simulink model "SHM_900HZ_TG190428test"  (Simulink 7.7)
settings: Solver=ode113  SolverMode=SingleTasking  StartTime=0.0  StopTime=3  RelTol=0.5e-4
undefined symbols (not defined in the file): D11, Delta, SHM900
libraries: powerlib x37, powerlib_extras x22, simulink x6, simulink_extras x1
(part 1 of 2)
settings Model: Creator=wufenglin  LastModifiedBy=jinxuefeng  SimulationMode=accelerator
settings SolverCC: AutoInsertRateTranBlk=on
settings OptimizationCC: InitFltsAndDblsToZero=on  EfficientMapNaN2IntZero=off
settings DebuggingCC: SaveWithParameterizedLinksMsg=none  SignalResolutionControl=TryResolveAllWithWarning  UnconnectedInputMsg=none  UnconnectedOutputMsg=none  UnconnectedLineMsg=none  StrictBusMsg=Warning
settings HardwareCC: TargetIntDivRoundTo=Zero  TargetEndianess=LittleEndian  TargetHWDeviceType=MATLAB Host  ProdEqTarget=off
settings CodeAppCC: MaxIdLength=128

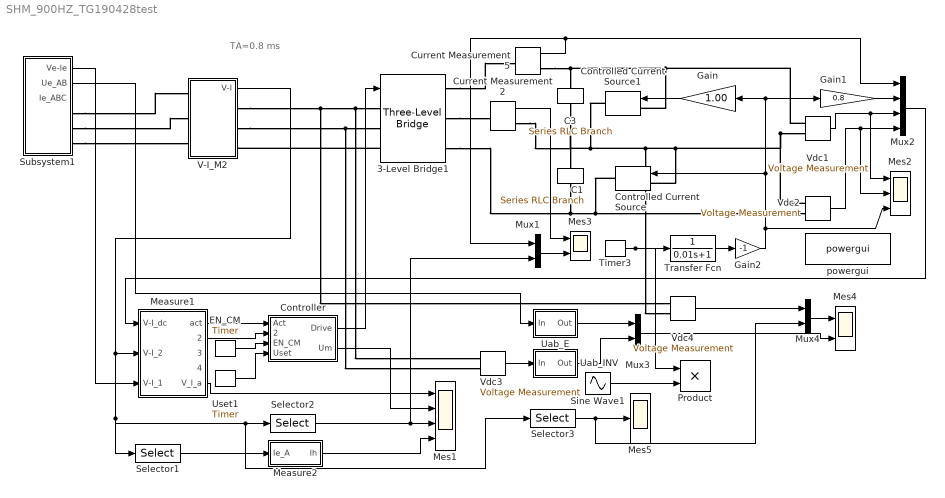
== system SHM_900HZ_TG190428test ==
  note: TA=0.8 ms
  3-Level Bridge1 : powerlib/Power Electronics/Three-Level Bridge  SystemSampleTime=-1  Arms=3  SnubberResistance=10000  SbubberCapacitance=1e-6  Device=MOSFET / Diodes  Ron=0.2e-3  ForwardVoltages="[  2 1 ]"  Measurements=None
  C1 : powerlib/Elements/Series RLC Branch  PhysicalDomain=powersysdomain  SubClassName=unknown  LeftPortType=p1  RightPortType=p1  LConnTagsString=__new0  RConnTagsString=__new0  BranchType=C  Resistance=1.0  Inductance=1.0  SetiL0=off  InitialCurrent=0  Capacitance=14e-3  Setx0=on  InitialVoltage=2600  Measurements=None
  C3 : powerlib/Elements/Series RLC Branch  PhysicalDomain=powersysdomain  SubClassName=unknown  LeftPortType=p1  RightPortType=p1  LConnTagsString=__new0  RConnTagsString=__new0  BranchType=C  Resistance=1.0  Inductance=1.0  SetiL0=off  InitialCurrent=0  Capacitance=14e-3  Setx0=on  InitialVoltage=2600  Measurements=None
  Controlled Current Source : powerlib/Electrical Sources/Controlled Current Source  SystemSampleTime=-1  Initialize=on  Source_Type=AC  Amplitude=0  Phase=0  Frequency=0  Measurements=None
  Controlled Current Source1 : powerlib/Electrical Sources/Controlled Current Source  SystemSampleTime=-1  Initialize=on  Source_Type=AC  Amplitude=0  Phase=0  Frequency=0  Measurements=None
  Controller : Subsystem  mask{Ts=1e-6, TA=1/1800, fn=50, Kp_v=3, Tn_v=0.2, Kp_I=0.1, Tn_I=0.05, K1=1.011, T1=0.005, Iq0=-0.278*0, La=0.23, Td=2.5e-5, U2=3.3, Kpre=5, Kp_v_scal=2}
      mask prompts: Ts "Ts [s]"; TA "TA [s]"; fn "fn [Hz]"; T1 "T1 [s]"
  Current Measurement2 : powerlib/Measurements/Current Measurement  SystemSampleTime=-1  PhasorSimulation=off  OutputType=Complex  PSBequivalent=0
  Current Measurement5 : powerlib/Measurements/Current Measurement  SystemSampleTime=-1  PhasorSimulation=off  OutputType=Complex  PSBequivalent=0
  EN_CM : powerlib_extras/Control  Blocks/Timer  SystemSampleTime=-1  t="[ 0  10]"  e="[1  1]"
  Gain : Gain  Gain=1.00
  Gain1 : Gain  Gain=0.8
  Gain2 : Gain  Gain=-1
  Measure1 : Subsystem  mask{Ts=1e-6, TA=1/1800, Sn=8, U1=10, U2=3.3, Udc=2.4}
      mask prompts: Ts "Ts [s}"; TA "TA [s]"; Sn "Sn [MVA]"; U1 "U1 [kV]"; U2 "U2 [kV]"; Udc "Udc [kV]"
  Measure2 : Subsystem
  Mes1 : Scope  NumInputPorts=4
      settings: YMin=-1.1~-5~-5~-5  YMax=1.1~5~5~5  SaveName=Vdc2  SampleInput=on  SampleTime=1e-5
  Mes2 : Scope  NumInputPorts=3
      settings: YMin=2399.85~2399.84~-5  YMax=2399.89~2399.89~5  SaveName=Vdc  DataFormat=Array  SampleInput=on  SampleTime=1e-5
  Mes3 : Scope  NumInputPorts=2
      settings: YMin=-1.1~-5  YMax=1.1~5  SaveName=Vdc1  DataFormat=Array  SampleInput=on  SampleTime=1e-5
  Mes4 : Scope  NumInputPorts=2
      settings: YMin=-1000~-5  YMax=4750~5  SaveName=Vdc4  DataFormat=Array  SampleInput=on  SampleTime=1e-5
  Mes5 : Scope
      settings: YMin=-1.1  YMax=1.1  SaveName=IA_SHM900  SampleInput=on  SampleTime=1e-5
  Mux1 : Mux  Inputs=2
  Mux2 : Mux
  Mux3 : Mux  Inputs=2
  Mux4 : Mux  Inputs=2
  Product : Product  RndMeth=Zero
  Selector1 : Selector  InputPortWidth=5  IndexOptions=Index vector (dialog)  Indices=3  OutputSizes=1
  Selector2 : Selector  InputPortWidth=5  IndexOptions=Index vector (dialog)  Indices=[3 4 5]  OutputSizes=1
  Selector3 : Selector  InputPortWidth=5  IndexOptions=Index vector (dialog)  Indices=3  OutputSizes=1
  Sine Wave1 : Sin  Amplitude=0.8  Frequency=4*pi  SampleTime=0
  Subsystem1 : Subsystem
  Timer3 : powerlib_extras/Control  Blocks/Timer  SystemSampleTime=-1  t="[ 0  0.6 1.1 1.3]"  e="[0  1200  1200 1200]"
  Transfer Fcn : TransferFcn  Denominator=[0.01 1]
  Uab_E : Subsystem  mask{Period=0.667e-3, buf=2048}
      mask prompts: Period "average period"; buf "buffer size"
  Uab_INV : Subsystem  mask{Period=0.667e-3, buf=2048}
      mask prompts: Period "average period"; buf "buffer size"
  Uset1 : powerlib_extras/Control  Blocks/Timer  SystemSampleTime=-1  t="[ 0  10]"  e="[1.08  1]"
  V-I_M2 : Subsystem
  Vdc{1..4} (4 alike) : powerlib/Measurements/Voltage Measurement  Tag=PoWeRsYsTeMmEaSuReMeNt  SystemSampleTime=-1  PhasorSimulation=off  OutputType=Magnitude  PSBequivalent=0
  powergui : powerlib/powergui  SystemSampleTime=-1  SimulationMode=Discrete  SampleTime=1e-6  frequency=60  SPID=off  DisableSnubberDevices=off  DisableRonSwitches=off  DisableVfSwitches=off  SwTol=0  Interpol=off  DisplayEquations=off  FunctionMessages=off  frequencyindice=0  Pbase=100e6  ErrMax=1e-4  Iterations=50  UnitsV=kV  UnitsW=MW  echomessages=off  HookPort=off  EnableUseOfTLC=off  x0status=blocks  RestoreLinks=warning  ResistiveCurrentMeasurement=off  Frange=[0:2:500]  Ylog=off  Xlog=on  ShowGrid=off  save=off  variable=ZData  structure=IA_SHM900  ZoomFFT=off  StartTime=0.6  cycles=20  DisplayStyle=1  fundamental=50  FreqAxis=on  MaxFrequency=2000  frequencyindicesteady=1  RmsSteady=1  display=off  Ts=0  methode=off
  wires:
  Vdc2/1 -> Mux2/4, Mes2/2
  Mux2/1 -> Measure1/1(V-I_dc)
  Vdc1/1 -> Mux2/3, Mes2/1
  Current Measurement5/1 -> Mux2/1, Mux1/1
  Measure1/1(act) -> Controller/1(Act)
  Transfer Fcn/1 -> Gain2/1
  Controller/1(Drive) -> 3-Level Bridge1/1
  Mux1/1 -> Mes3/2
  Current Measurement2/1 -> Mes3/1
  V-I_M2/1(V-I) -> Measure1/2(V-I_2), Selector1/1, Selector2/1, Selector3/1
  Measure1/5(V_I_a) -> Mes1/1
  Uab_E/1(Out) -> Mux3/1
  Uab_INV/1(Out) -> Mux3/2
  Vdc3/1 -> Uab_INV/1(In)
  Measure1/2(Vdc_sub) -> Controller/2(Udc_sub)
  Gain/1 -> Controlled Current Source1/1
  EN_CM/1 -> Controller/3(EN_CM)
  Selector2/1 -> Mes1/3, Mux1/2
  Subsystem1/1(Ve-Ie) -> Measure1/3(V-I_1)
  Subsystem1/2(Ue_AB) -> Uab_E/1(In)
  Measure2/1(Ih) -> Mes1/4
  Selector1/1 -> Measure2/1(Ie_A)
  Selector3/1 -> Mes5/1, Mux4/2
  Controller/2(Um) -> Mes1/2
  Mux3/1 -> Mes4/2
  Uset1/1 -> Controller/4(Uset)
  Timer3/1 -> Product/1, Transfer Fcn/1
  Vdc4/1 -> Mux4/1
  Mux4/1 -> Mes4/1
  Gain1/1 -> Mux2/2
  Sine Wave1/1 -> Product/2
  Gain2/1 -> Controlled Current Source/1, Gain/1, Gain1/1, Mes2/3
  connections:
  Vdc1/LConn1 -- Current Measurement5/RConn1 -- C3/LConn1 -- Controlled Current Source1/LConn1
  3-Level Bridge1/RConn1 -- Current Measurement5/LConn1
  V-I_M2/RConn1 -- 3-Level Bridge1/LConn1 -- Vdc3/LConn1 -- Vdc4/LConn1
  V-I_M2/RConn2 -- 3-Level Bridge1/LConn2 -- Vdc3/LConn2
  3-Level Bridge1/LConn3 -- V-I_M2/RConn3
  3-Level Bridge1/RConn2 -- Current Measurement2/LConn1
  Vdc2/LConn1 -- Vdc1/LConn2 -- Controlled Current Source/LConn1 -- Current Measurement2/RConn1 -- C1/LConn1 -- C3/RConn1 -- Controlled Current Source1/RConn1 -- Vdc4/LConn2
  3-Level Bridge1/RConn3 -- C1/RConn1 -- Vdc2/LConn2 -- Controlled Current Source/RConn1
  Subsystem1/RConn3 -- V-I_M2/LConn3
  Subsystem1/RConn2 -- V-I_M2/LConn2
  Subsystem1/RConn1 -- V-I_M2/LConn1

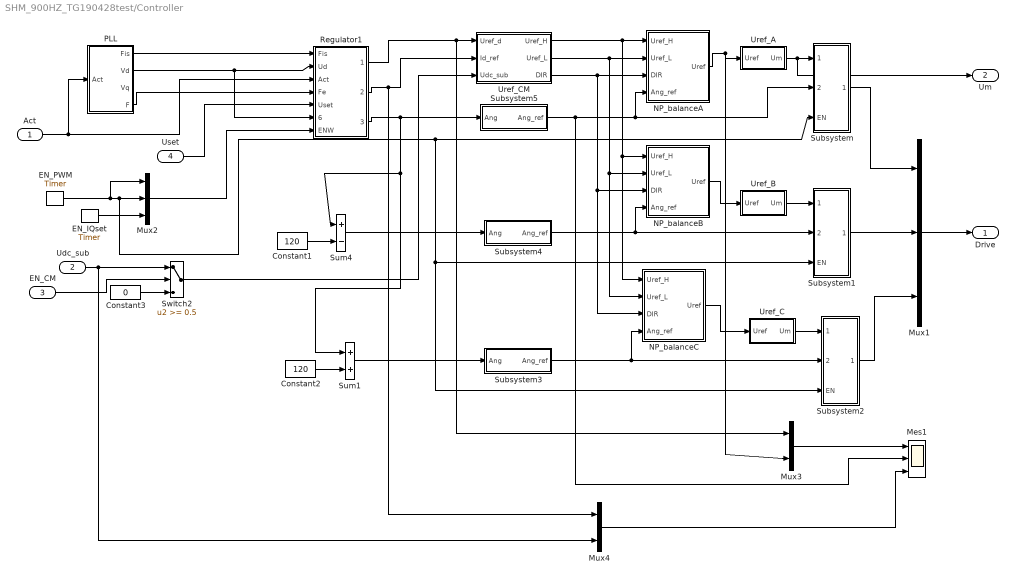
== system SHM_900HZ_TG190428test/Controller ==
  Act : Inport
  Udc_sub : Inport  Port=2
  EN_CM : Inport  Port=3
  Uset : Inport  Port=4
  Constant1 : Constant  Value=120
  Constant2 : Constant  Value=120
  Constant3 : Constant  Value=0
  EN_IQset : powerlib_extras/Control  Blocks/Timer  SystemSampleTime=-1  t="[ 0    0.16  0.22 ]"  e="[  0  1  1]"
  EN_PWM : powerlib_extras/Control  Blocks/Timer  SystemSampleTime=-1  t="[ 0    0.1 ]"  e="[  0  1 ]"
  Mes1 : Scope  NumInputPorts=3
      settings: YMin=-1.1~-5~-5  YMax=1.1~5~5  SaveName=Vdc6  SampleInput=on  SampleTime=1e-5
  Mux1 : Mux  Inputs=3
  Mux2 : Mux  Inputs=3
  Mux3 : Mux  Inputs=2
  Mux4 : Mux  Inputs=2
  NP_balanceA : Subsystem
  NP_balanceB : Subsystem
  NP_balanceC : Subsystem
  PLL : Subsystem
  Regulator1 : Subsystem
  Subsystem : Subsystem
  Subsystem1 : Subsystem
  Subsystem2 : Subsystem
  Subsystem3 : Subsystem
  Subsystem4 : Subsystem
  Subsystem5 : Subsystem
  Sum1 : Sum  SampleTime=Ts
  Sum4 : Sum  Inputs=+-  SampleTime=Ts
  Switch2 : Switch  Threshold=0.5  ZeroCross=off  SampleTime=TA
  Uref_A : Subsystem
  Uref_B : Subsystem
  Uref_C : Subsystem
  Uref_CM : Subsystem
  Drive : Outport
  Um : Outport  Port=2
  wires:
  PLL/2(Vd) -> Regulator1/2(Ud), Regulator1/6(Ud_net)
  PLL/1(Fis) -> Regulator1/1(Fis)
  Act/1 -> PLL/1(Act), Regulator1/3(Act)
  PLL/4(F) -> Regulator1/4(Fe)
  Regulator1/3(Angle_d) -> Sum4/1, Sum1/1, Subsystem5/1(Ang)
  Constant1/1 -> Sum4/2
  Constant2/1 -> Sum1/2
  Sum4/1 -> Subsystem4/1(Ang)
  Sum1/1 -> Subsystem3/1(Ang)
  Subsystem/1(Puls) -> Mux1/1
  Subsystem1/1(Puls) -> Mux1/2
  Subsystem2/1(Puls) -> Mux1/3
  Mux1/1 -> Drive/1
  EN_PWM/1 -> Mux2/2, Subsystem/3(EN), Subsystem2/3(EN), Subsystem1/3(EN), Mux2/1
  EN_IQset/1 -> Mux2/3
  Mux2/1 -> Regulator1/7(ENW)
  Subsystem5/1(Ang_ref) -> Subsystem/2(Ang), NP_balanceA/4(Ang_ref), Mes1/2
  Subsystem4/1(Ang_ref) -> Subsystem1/2(Ang), NP_balanceB/4(Ang_ref)
  Subsystem3/1(Ang_ref) -> Subsystem2/2(Ang), NP_balanceC/4(Ang_ref)
  Uref_A/1(Um) -> Subsystem/1(U_d), Um/1
  NP_balanceA/1(Uref) -> Uref_A/1(Uref), Mux3/2
  NP_balanceB/1(Uref) -> Uref_B/1(Uref)
  Uref_B/1(Um) -> Subsystem1/1(U_d)
  Uref_C/1(Um) -> Subsystem2/1(U_d)
  NP_balanceC/1(Uref) -> Uref_C/1(Uref)
  Regulator1/1(Uref_d) -> Uref_CM/1(Uref_d), Mux3/1
  Regulator1/2(Id_ref) -> Uref_CM/2(Id_ref), Mux4/1
  Udc_sub/1 -> Switch2/1, Mux4/2
  Uref_CM/1(Uref_H) -> NP_balanceA/1(Uref_H), NP_balanceB/1(Uref_H), NP_balanceC/1(Uref_H)
  Uref_CM/2(Uref_L) -> NP_balanceA/2(Uref_L), NP_balanceB/2(Uref_L), NP_balanceC/2(Uref_L)
  Uref_CM/3(DIR) -> NP_balanceA/3(DIR), NP_balanceB/3(DIR), NP_balanceC/3(DIR)
  Mux3/1 -> Mes1/1
  Mux4/1 -> Mes1/3
  Switch2/1 -> Uref_CM/3(Udc_sub)
  Constant3/1 -> Switch2/3
  EN_CM/1 -> Switch2/2
  Uset/1 -> Regulator1/5(Uset)

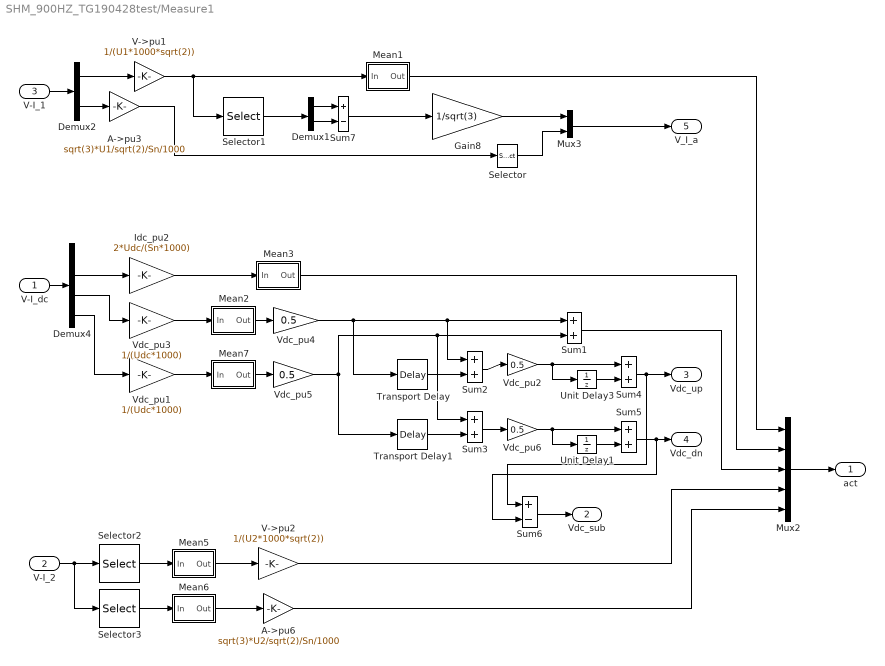
== system SHM_900HZ_TG190428test/Measure1 ==
  V-I_dc : Inport
  V-I_2 : Inport  Port=2
  V-I_1 : Inport  Port=3
  A->pu3 : Gain  Gain=sqrt(3)*U1/sqrt(2)/Sn/1000  SampleTime=Ts  SaturateOnIntegerOverflow=on  OutDataTypeStr=Inherit: Same as input  ParamDataTypeStr=Inherit: Same as input
  A->pu6 : Gain  Gain=sqrt(3)*U2/sqrt(2)/Sn/1000  SampleTime=Ts  SaturateOnIntegerOverflow=on  OutDataTypeStr=Inherit: Same as input  ParamDataTypeStr=Inherit: Same as input
  Demux1 : Demux  Outputs=2
  Demux2 : Demux  Outputs=2
  Demux4 : Demux
  Gain8 : Gain  Gain=1/sqrt(3)  SampleTime=Ts
  Idc_pu2 : Gain  Gain=2*Udc/(Sn*1000)  SampleTime=Ts  SaturateOnIntegerOverflow=on  OutDataTypeStr=Inherit: Same as input  ParamDataTypeStr=Inherit: Same as input
  Mean1 : Subsystem  mask{Period=TA, buf=2048}
      mask prompts: Period "average period"; buf "buffer size"
  Mean2 : Subsystem  mask{Period=TA, buf=2048}
      mask prompts: Period "average period"; buf "buffer size"
  Mean3 : Subsystem  mask{Period=TA, buf=2048}
      mask prompts: Period "average period"; buf "buffer size"
  Mean5 : Subsystem  mask{Period=TA, buf=2048}
      mask prompts: Period "average period"; buf "buffer size"
  Mean6 : Subsystem  mask{Period=TA, buf=2048}
      mask prompts: Period "average period"; buf "buffer size"
  Mean7 : Subsystem  mask{Period=TA, buf=2048}
      mask prompts: Period "average period"; buf "buffer size"
  Mux2 : Mux  Inputs=5
  Mux3 : Mux  Inputs=2
  Selector : Selector  InputPortWidth=3  IndexOptions=Index vector (dialog)  Indices=1  OutputSizes=1
  Selector1 : Selector  InputPortWidth=3  IndexOptions=Index vector (dialog)  Indices=[1 3]  OutputSizes=1
  Selector2 : Selector  InputPortWidth=5  IndexOptions=Index vector (dialog)  Indices=[1 2]  OutputSizes=1
  Selector3 : Selector  InputPortWidth=5  IndexOptions=Index vector (dialog)  Indices=[3 4 5]  OutputSizes=1
  Sum{1..5} (5 alike) : Sum  SampleTime=TA  SaturateOnIntegerOverflow=on  InputSameDT=on  OutDataTypeStr=Inherit: Same as first input
  Sum6 : Sum  Inputs=+-  SampleTime=TA  SaturateOnIntegerOverflow=on  InputSameDT=on  OutDataTypeStr=Inherit: Same as first input
  Sum7 : Sum  Inputs=+-  SampleTime=Ts
  Transport Delay : TransportDelay  DelayTime=3.445e-3
  Transport Delay1 : TransportDelay  DelayTime=3.445e-3
  Unit Delay1 : UnitDelay  SampleTime=TA
  Unit Delay3 : UnitDelay  SampleTime=TA
  V->pu1 : Gain  Gain=1/(U1*1000*sqrt(2))  SampleTime=Ts  SaturateOnIntegerOverflow=on  OutDataTypeStr=Inherit: Same as input  ParamDataTypeStr=Inherit: Same as input
  V->pu2 : Gain  Gain=1/(U2*1000*sqrt(2))  SampleTime=Ts  SaturateOnIntegerOverflow=on  OutDataTypeStr=Inherit: Same as input  ParamDataTypeStr=Inherit: Same as input
  Vdc_pu1 : Gain  Gain=1/(Udc*1000)  SampleTime=Ts  SaturateOnIntegerOverflow=on  OutDataTypeStr=Inherit: Same as input  ParamDataTypeStr=Inherit: Same as input
  Vdc_pu{2,4..6} (4 alike) : Gain  Gain=0.5  SampleTime=TA  SaturateOnIntegerOverflow=on  OutDataTypeStr=Inherit: Same as input  ParamDataTypeStr=Inherit: Same as input
  Vdc_pu3 : Gain  Gain=1/(Udc*1000)  SampleTime=Ts  SaturateOnIntegerOverflow=on  OutDataTypeStr=Inherit: Same as input  ParamDataTypeStr=Inherit: Same as input
  act : Outport
  Vdc_sub : Outport  Port=2
  Vdc_up : Outport  Port=3
  Vdc_dn : Outport  Port=4
  V_I_a : Outport  Port=5
  wires:
  Idc_pu2/1 -> Mean3/1(In)
  Vdc_pu3/1 -> Mean2/1(In)
  Demux2/1 -> V->pu1/1
  Demux2/2 -> A->pu3/1
  V->pu1/1 -> Selector1/1, Mean1/1(In)
  V-I_1/1 -> Demux2/1
  Sum7/1 -> Gain8/1
  Selector1/1 -> Demux1/1
  Demux1/1 -> Sum7/1
  Demux1/2 -> Sum7/2
  A->pu3/1 -> Selector/1
  Sum1/1 -> Mux2/3
  Vdc_pu1/1 -> Mean7/1(In)
  Mean1/1(Out) -> Mux2/1
  Mean3/1(Out) -> Mux2/2
  V-I_dc/1 -> Demux4/1
  Demux4/2 -> Idc_pu2/1
  Demux4/3 -> Vdc_pu3/1
  Demux4/4 -> Vdc_pu1/1
  V-I_2/1 -> Selector2/1, Selector3/1
  Selector2/1 -> Mean5/1(In)
  Selector3/1 -> Mean6/1(In)
  A->pu6/1 -> Mux2/5
  V->pu2/1 -> Mux2/4
  Mux2/1 -> act/1
  Mean5/1(Out) -> V->pu2/1
  Mean6/1(Out) -> A->pu6/1
  Gain8/1 -> Mux3/1
  Selector/1 -> Mux3/2
  Mux3/1 -> V_I_a/1
  Mean2/1(Out) -> Vdc_pu4/1
  Mean7/1(Out) -> Vdc_pu5/1
  Vdc_pu4/1 -> Transport Delay/1, Sum1/1, Sum2/1
  Vdc_pu5/1 -> Transport Delay1/1, Sum1/2, Sum3/1
  Transport Delay/1 -> Sum2/2
  Sum2/1 -> Vdc_pu2/1
  Unit Delay3/1 -> Sum4/2
  Vdc_pu2/1 -> Sum4/1, Unit Delay3/1
  Transport Delay1/1 -> Sum3/2
  Sum3/1 -> Vdc_pu6/1
  Unit Delay1/1 -> Sum5/2
  Vdc_pu6/1 -> Sum5/1, Unit Delay1/1
  Sum4/1 -> Vdc_up/1, Sum6/1
  Sum5/1 -> Vdc_dn/1, Sum6/2
  Sum6/1 -> Vdc_sub/1

== system SHM_900HZ_TG190428test/Measure2 ==
  Ie_A : Inport
  Saturation1 : Saturate  UpperLimit=0.2  LowerLimit=-0.1  ZeroCross=off
  Total Harmonic Distorsion1 : powerlib_extras/Measurements/Total Harmonic Distortion  SystemSampleTime=-1  f1=50
  Ih : Outport
  wires:
  Total Harmonic Distorsion1/1 -> Saturation1/1
  Saturation1/1 -> Ih/1
  Ie_A/1 -> Total Harmonic Distorsion1/1

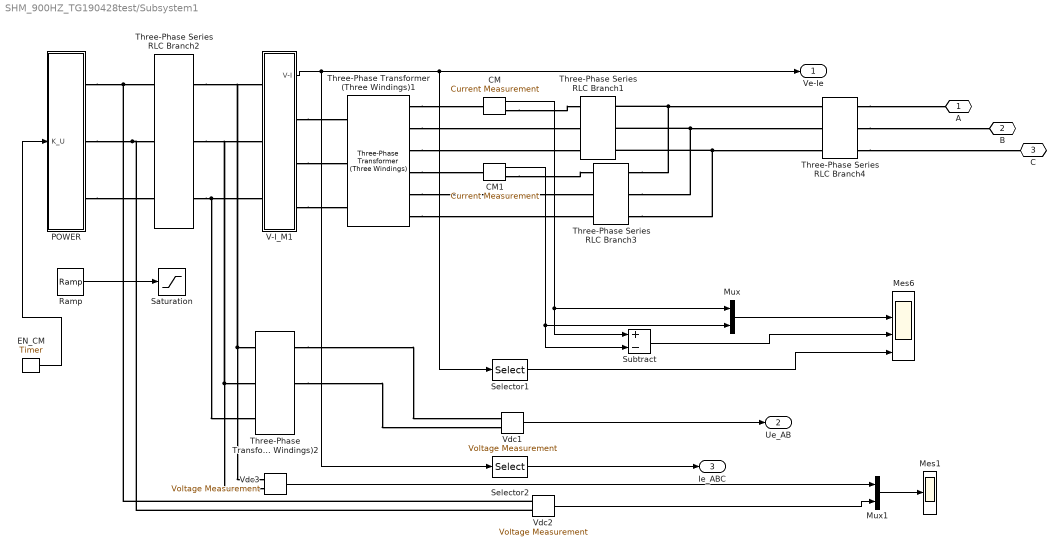
== system SHM_900HZ_TG190428test/Subsystem1 ==
  CM : powerlib/Measurements/Current Measurement  SystemSampleTime=-1  PhasorSimulation=off  OutputType=Complex  PSBequivalent=0
  CM1 : powerlib/Measurements/Current Measurement  SystemSampleTime=-1  PhasorSimulation=off  OutputType=Complex  PSBequivalent=0
  EN_CM : powerlib_extras/Control  Blocks/Timer  SystemSampleTime=-1  t="[ 0  1.5 1.6]"  e="[1  1.1 1]"
  Mes1 : Scope
      settings: YMin=4710  YMax=4910  SaveName=Vdc3  DataFormat=Array  SampleInput=on  SampleTime=1e-5
  Mes6 : Scope  NumInputPorts=4
      settings: YMin=4710~-1~-5~-5  YMax=4910~1~5~5  SaveName=Vdc9  DataFormat=Array  SampleInput=on  SampleTime=1e-5
  Mux : Mux  Inputs=2
  Mux1 : Mux  Inputs=2
  POWER : Subsystem  mask{UL=10, Uth=0, TH=13}
      mask prompts: UL "UL(kV)"; Uth "Uth(pu)"; TH "TH(fn)"
  Ramp : simulink/Sources/Ramp  SystemSampleTime=-1  slope=0.1  start=0.6  X0=0.9
  Saturation : Saturate  UpperLimit=1.04  LowerLimit=0.9
  Selector1 : Selector  InputPortWidth=6  IndexOptions=Index vector (dialog)  Indices=[4]  OutputSizes=1
  Selector2 : Selector  InputPortWidth=6  IndexOptions=Index vector (dialog)  Indices=[4 5 6]  OutputSizes=1
  Subtract : Sum  Inputs=+-
  Three-Phase Series RLC Branch1 : powerlib/Elements/Three-Phase Series RLC Branch  PhysicalDomain=powersysdomain  SubClassName=unknown  LeftPortType=p1  RightPortType=p1  LConnTagsString=A|B|C  RConnTagsString=A|B|C  BranchType=L  Resistance=0.01  Inductance=0.45e-3  Capacitance=1e-6  Measurements=None
  Three-Phase Series RLC Branch2 : powerlib/Elements/Three-Phase Series RLC Branch  PhysicalDomain=powersysdomain  SubClassName=unknown  LeftPortType=p1  RightPortType=p1  LConnTagsString=A|B|C  RConnTagsString=A|B|C  BranchType=RL  Resistance=0.01  Inductance=0.5e-3  Capacitance=1e-6  Measurements=None
  Three-Phase Series RLC Branch3 : powerlib/Elements/Three-Phase Series RLC Branch  PhysicalDomain=powersysdomain  SubClassName=unknown  LeftPortType=p1  RightPortType=p1  LConnTagsString=A|B|C  RConnTagsString=A|B|C  BranchType=L  Resistance=0.01  Inductance=0.45e-3  Capacitance=1e-6  Measurements=None
  Three-Phase Series RLC Branch4 : powerlib/Elements/Three-Phase Series RLC Branch  PhysicalDomain=powersysdomain  SubClassName=unknown  LeftPortType=p1  RightPortType=p1  LConnTagsString=A|B|C  RConnTagsString=A|B|C  BranchType=L  Resistance=0.01  Inductance=0.6e-3  Capacitance=1e-6  Measurements=None
  Three-Phase Transformer (Three Windings)1 : powerlib/Elements/Three-Phase Transformer (Three Windings)  SystemSampleTime=-1  Winding1Connection=Delta (D11)  UNITS=pu  NominalPower=[ 8e6 , 50 ]  Winding1=[ 10e3 , 0.002 , 0.04 ]  Winding2Connection=Y  Winding2=[ 3.4e3 , 0.002 , 0.039 ]  Winding3Connection=Y  Winding3=[ 3.4e3 , 0.002 , 0.041 ]  SetSaturation=off  Rm=500  Lm=500  Saturation=[ 0,0 ; 0.0024,1.2 ; 1.0,1.52 ]  Hysteresis=off  DataFile='hysteresis'  SetInitialFlux=off  InitialFluxes=[0.8 -0.8 0.7]  Measurements=None  MoreParameters=off  BreakLoop=off  DataType=off  TransfoNumber=1
  Three-Phase Transformer (Two Windings)2 : powerlib/Elements/Three-Phase Transformer (Two Windings)  SystemSampleTime=-1  Winding1Connection=Delta (D11)  UNITS=pu  NominalPower=[ 8e6 , 50 ]  Winding1=[ 10e3 , 0.002 , 0.04]  Winding2Connection=Y  Winding2=[ 3e3 , 0.002 , 0.04 ]  SetSaturation=off  Rm=500  Lm=500  Saturation=[ 0,0 ; 0.0024,1.2 ; 1.0,1.52 ]  Hysteresis=off  DataFile='hysteresis'  SetInitialFlux=off  InitialFluxes=[ 0.8 , -0.8 , 0.7 ]  Measurements=None  MoreParameters=off  BreakLoop=off  DataType=off  TransfoNumber=0
  V-I_M1 : Subsystem
  Vdc1 : powerlib/Measurements/Voltage Measurement  Tag=PoWeRsYsTeMmEaSuReMeNt  SystemSampleTime=-1  PhasorSimulation=off  OutputType=Magnitude  PSBequivalent=0
  Vdc2 : powerlib/Measurements/Voltage Measurement  Tag=PoWeRsYsTeMmEaSuReMeNt  SystemSampleTime=-1  PhasorSimulation=off  OutputType=Magnitude  PSBequivalent=0
  Vdc3 : powerlib/Measurements/Voltage Measurement  Tag=PoWeRsYsTeMmEaSuReMeNt  SystemSampleTime=-1  PhasorSimulation=off  OutputType=Magnitude  PSBequivalent=0
  A : PMIOPort  Port=1  Side=Right
  B : PMIOPort  Port=2  Side=Right
  C : PMIOPort  Port=3  Side=Right
  Ve-Ie : Outport
  Ue_AB : Outport  Port=2
  Ie_ABC : Outport  Port=3
  wires:
  V-I_M1/1(V-I) -> Ve-Ie/1, Selector1/1, Selector2/1
  Mux/1 -> Mes6/2
  Subtract/1 -> Mes6/3
  Selector1/1 -> Mes6/4
  CM/1 -> Subtract/1, Mux/1
  CM1/1 -> Subtract/2, Mux/2
  Vdc1/1 -> Ue_AB/1
  Selector2/1 -> Ie_ABC/1
  Vdc2/1 -> Mux1/2
  Mux1/1 -> Mes1/1
  Ramp/1 -> Saturation/1
  Vdc3/1 -> Mux1/1
  EN_CM/1 -> POWER/1(K_U)
  connections:
  Three-Phase Transformer (Three Windings)1/RConn3 -- Three-Phase Series RLC Branch1/LConn3
  Three-Phase Transformer (Three Windings)1/RConn2 -- Three-Phase Series RLC Branch1/LConn2
  Three-Phase Series RLC Branch3/RConn1 -- Three-Phase Series RLC Branch1/RConn1 -- Three-Phase Series RLC Branch4/LConn1
  Three-Phase Series RLC Branch3/RConn2 -- Three-Phase Series RLC Branch1/RConn2 -- Three-Phase Series RLC Branch4/LConn2
  Three-Phase Series RLC Branch3/RConn3 -- Three-Phase Series RLC Branch1/RConn3 -- Three-Phase Series RLC Branch4/LConn3
  V-I_M1/RConn1 -- Three-Phase Transformer (Three Windings)1/LConn1
  V-I_M1/RConn2 -- Three-Phase Transformer (Three Windings)1/LConn2
  V-I_M1/RConn3 -- Three-Phase Transformer (Three Windings)1/LConn3
  Three-Phase Transformer (Three Windings)1/RConn1 -- CM/LConn1
  Three-Phase Transformer (Three Windings)1/RConn4 -- CM1/LConn1
  Three-Phase Series RLC Branch2/RConn2 -- V-I_M1/LConn2 -- Three-Phase Transformer (Two Windings)2/LConn2 -- Vdc3/LConn2
  Three-Phase Series RLC Branch2/RConn3 -- V-I_M1/LConn3 -- Three-Phase Transformer (Two Windings)2/LConn3
  Three-Phase Series RLC Branch2/RConn1 -- V-I_M1/LConn1 -- Three-Phase Transformer (Two Windings)2/LConn1 -- Vdc3/LConn1
  Three-Phase Transformer (Two Windings)2/RConn1 -- Vdc1/LConn1
  Three-Phase Transformer (Two Windings)2/RConn2 -- Vdc1/LConn2
  Vdc2/LConn1 -- Three-Phase Series RLC Branch2/LConn1 -- POWER/RConn1
  Vdc2/LConn2 -- Three-Phase Series RLC Branch2/LConn2 -- POWER/RConn2
  POWER/RConn3 -- Three-Phase Series RLC Branch2/LConn3
  CM/RConn1 -- Three-Phase Series RLC Branch1/LConn1
  CM1/RConn1 -- Three-Phase Series RLC Branch3/LConn1
  Three-Phase Transformer (Three Windings)1/RConn5 -- Three-Phase Series RLC Branch3/LConn2
  Three-Phase Transformer (Three Windings)1/RConn6 -- Three-Phase Series RLC Branch3/LConn3
  Three-Phase Series RLC Branch4/RConn1 -- A/RConn1
  Three-Phase Series RLC Branch4/RConn2 -- B/RConn1
  Three-Phase Series RLC Branch4/RConn3 -- C/RConn1

== system SHM_900HZ_TG190428test/Uab_E ==
  In : Inport
  Gain : Gain  Gain=1/Period  SaturateOnIntegerOverflow=on  OutDataTypeStr=Inherit: Same as input  ParamDataTypeStr=Inherit: Same as input
  Integrator : Integrator
  Sum : Sum  Inputs=+-  SaturateOnIntegerOverflow=on  InputSameDT=on  OutDataTypeStr=Inherit: Same as first input
  Transport Delay : TransportDelay  DelayTime=Period  BufferSize=buf
  Out : Outport
  wires:
  Gain/1 -> Out/1
  Integrator/1 -> Sum/1, Transport Delay/1
  In/1 -> Integrator/1
  Transport Delay/1 -> Sum/2
  Sum/1 -> Gain/1

== system SHM_900HZ_TG190428test/Uab_INV ==
  In : Inport
  Gain : Gain  Gain=1/Period  SaturateOnIntegerOverflow=on  OutDataTypeStr=Inherit: Same as input  ParamDataTypeStr=Inherit: Same as input
  Integrator : Integrator
  Sum : Sum  Inputs=+-  SaturateOnIntegerOverflow=on  InputSameDT=on  OutDataTypeStr=Inherit: Same as first input
  Transport Delay : TransportDelay  DelayTime=Period  BufferSize=buf
  Out : Outport
  wires:
  Sum/1 -> Gain/1
  Transport Delay/1 -> Sum/2
  In/1 -> Integrator/1
  Integrator/1 -> Transport Delay/1, Sum/1
  Gain/1 -> Out/1

== system SHM_900HZ_TG190428test/V-I_M2 ==
  CM : powerlib/Measurements/Current Measurement  SystemSampleTime=-1  PhasorSimulation=off  OutputType=Complex  PSBequivalent=0
  CM1 : powerlib/Measurements/Current Measurement  SystemSampleTime=-1  PhasorSimulation=off  OutputType=Complex  PSBequivalent=0
  CM2 : powerlib/Measurements/Current Measurement  SystemSampleTime=-1  PhasorSimulation=off  OutputType=Complex  PSBequivalent=0
  Mes3 : Scope  NumInputPorts=2
      settings: YMin=-1.1~-5  YMax=1.1~5  SaveName=Vdc5  DataFormat=Array  SampleInput=on  SampleTime=1e-5
  Mux4 : Mux  Inputs=5
  Vab : powerlib/Measurements/Voltage Measurement  Tag=PoWeRsYsTeMmEaSuReMeNt  SystemSampleTime=-1  PhasorSimulation=off  OutputType=Magnitude  PSBequivalent=0
  Vab1 : powerlib/Measurements/Voltage Measurement  Tag=PoWeRsYsTeMmEaSuReMeNt  SystemSampleTime=-1  PhasorSimulation=off  OutputType=Magnitude  PSBequivalent=0
  In1 : PMIOPort  Port=1  Side=Left
  In2 : PMIOPort  Port=2  Side=Left
  In3 : PMIOPort  Port=3  Side=Left
  Out1 : PMIOPort  Port=4  Side=Right
  Out2 : PMIOPort  Port=5  Side=Right
  Out3 : PMIOPort  Port=6  Side=Right
  V-I : Outport
  wires:
  CM1/1 -> Mux4/5
  CM2/1 -> Mux4/4, Mes3/1
  CM/1 -> Mux4/3, Mes3/2
  Mux4/1 -> V-I/1
  Vab1/1 -> Mux4/2
  Vab/1 -> Mux4/1
  connections:
  CM2/LConn1 -- In2/RConn1 -- Vab/LConn2 -- Vab1/LConn1
  CM1/LConn1 -- In3/RConn1 -- Vab1/LConn2
  CM/LConn1 -- In1/RConn1 -- Vab/LConn1
  Out1/RConn1 -- CM/RConn1
  Out2/RConn1 -- CM2/RConn1
  Out3/RConn1 -- CM1/RConn1

== system SHM_900HZ_TG190428test/Controller/NP_balanceA ==
  Uref_H : Inport
  Uref_L : Inport  Port=2
  DIR : Inport  Port=3
  Ang_ref : Inport  Port=4
  Constant4 : Constant  Value=180
  Logical Operator : Logic  Operator=XOR  AllPortsSameDT=off  OutDataTypeStr=boolean
  Relational Operator1 : RelationalOperator  Operator=<=  OutDataTypeStr=boolean  SampleTime=TA
  Switch2 : Switch  Threshold=0.5  ZeroCross=off  SampleTime=TA
  Uref : Outport
  wires:
  DIR/1 -> Logical Operator/2
  Constant4/1 -> Relational Operator1/2
  Uref_H/1 -> Switch2/3
  Uref_L/1 -> Switch2/1
  Ang_ref/1 -> Relational Operator1/1
  Relational Operator1/1 -> Logical Operator/1
  Logical Operator/1 -> Switch2/2
  Switch2/1 -> Uref/1

== system SHM_900HZ_TG190428test/Controller/NP_balanceB ==
  Uref_H : Inport
  Uref_L : Inport  Port=2
  DIR : Inport  Port=3
  Ang_ref : Inport  Port=4
  Constant4 : Constant  Value=180
  Logical Operator : Logic  Operator=XOR  AllPortsSameDT=off  OutDataTypeStr=boolean
  Relational Operator1 : RelationalOperator  Operator=<=  OutDataTypeStr=boolean  SampleTime=TA
  Switch2 : Switch  Threshold=0.5  ZeroCross=off  SampleTime=TA
  Uref : Outport
  wires:
  Switch2/1 -> Uref/1
  Logical Operator/1 -> Switch2/2
  Relational Operator1/1 -> Logical Operator/1
  Ang_ref/1 -> Relational Operator1/1
  Uref_L/1 -> Switch2/1
  Uref_H/1 -> Switch2/3
  Constant4/1 -> Relational Operator1/2
  DIR/1 -> Logical Operator/2

== system SHM_900HZ_TG190428test/Controller/NP_balanceC ==
  Uref_H : Inport
  Uref_L : Inport  Port=2
  DIR : Inport  Port=3
  Ang_ref : Inport  Port=4
  Constant4 : Constant  Value=180
  Logical Operator : Logic  Operator=XOR  AllPortsSameDT=off  OutDataTypeStr=boolean
  Relational Operator1 : RelationalOperator  Operator=<=  OutDataTypeStr=boolean  SampleTime=TA
  Switch2 : Switch  Threshold=0.5  ZeroCross=off  SampleTime=TA
  Uref : Outport
  wires:
  DIR/1 -> Logical Operator/2
  Constant4/1 -> Relational Operator1/2
  Uref_H/1 -> Switch2/3
  Uref_L/1 -> Switch2/1
  Ang_ref/1 -> Relational Operator1/1
  Relational Operator1/1 -> Logical Operator/1
  Logical Operator/1 -> Switch2/2
  Switch2/1 -> Uref/1

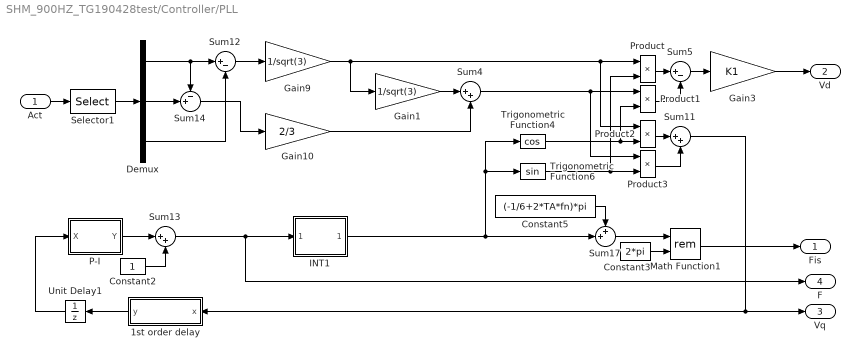
== system SHM_900HZ_TG190428test/Controller/PLL ==
  Act : Inport
  1st order delay : Subsystem
  Constant2 : Constant
  Constant3 : Constant  Value=2*pi
  Constant5 : Constant  Value=(-1/6+2*TA*fn)*pi
  Demux : Demux  Outputs=3
  Gain1 : Gain  Gain=1/sqrt(3)  SampleTime=TA
  Gain10 : Gain  Gain=2/3  SampleTime=TA
  Gain3 : Gain  Gain=K1  SampleTime=TA
  Gain9 : Gain  Gain=1/sqrt(3)  SampleTime=TA
  INT1 : Subsystem
  Math Function1 : Math  Operator=rem  SampleTime=TA  SaturateOnIntegerOverflow=on
  P-I : Subsystem
  Product{,1..3} (4 alike) : Product  SampleTime=TA  RndMeth=Zero
  Selector1 : Selector  InputPortWidth=10  IndexOptions=Index vector (dialog)  Indices=[1 2 3]  OutputSizes=1
  Sum11 : Sum  Inputs=|++  SampleTime=TA
  Sum12 : Sum  Inputs=|+-  SampleTime=TA
  Sum13 : Sum  Inputs=|++  SampleTime=TA
  Sum14 : Sum  Inputs=-+|  SampleTime=TA
  Sum17 : Sum  Inputs=++|  SampleTime=TA
  Sum4 : Sum  Inputs=|++  SampleTime=TA
  Sum5 : Sum  Inputs=|+-  SampleTime=TA
  Trigonometric Function4 : Trigonometry  Operator=cos  SampleTime=TA
  Trigonometric Function6 : Trigonometry  SampleTime=TA
  Unit Delay1 : UnitDelay  SampleTime=TA
  Fis : Outport
  Vd : Outport  Port=2
  Vq : Outport  Port=3
  F : Outport  Port=4
  wires:
  Constant5/1 -> Sum17/1
  Sum17/1 -> Math Function1/1
  Sum14/1 -> Gain10/1
  Sum12/1 -> Gain9/1
  Gain9/1 -> Gain1/1, Product/1, Product2/1
  Demux/2 -> Sum14/2
  Demux/1 -> Sum14/1, Sum12/1
  Gain1/1 -> Sum4/1
  Trigonometric Function4/1 -> Product1/2, Product2/2
  Trigonometric Function6/1 -> Product/2, Product3/2
  Sum4/1 -> Product1/1, Product3/1
  Product/1 -> Sum5/1
  Product1/1 -> Sum5/2
  Product2/1 -> Sum11/1
  Product3/1 -> Sum11/2
  Constant2/1 -> Sum13/2
  Sum13/1 -> INT1/1(Freq), F/1
  Sum11/1 -> 1st order delay/1(x), Vq/1
  Sum5/1 -> Gain3/1
  INT1/1(Angle) -> Trigonometric Function6/1, Trigonometric Function4/1, Sum17/2
  Demux/3 -> Sum12/2
  Unit Delay1/1 -> P-I/1(X)
  P-I/1(Y) -> Sum13/1
  1st order delay/1(y) -> Unit Delay1/1
  Gain10/1 -> Sum4/2
  Gain3/1 -> Vd/1
  Act/1 -> Selector1/1
  Selector1/1 -> Demux/1
  Constant3/1 -> Math Function1/2
  Math Function1/1 -> Fis/1

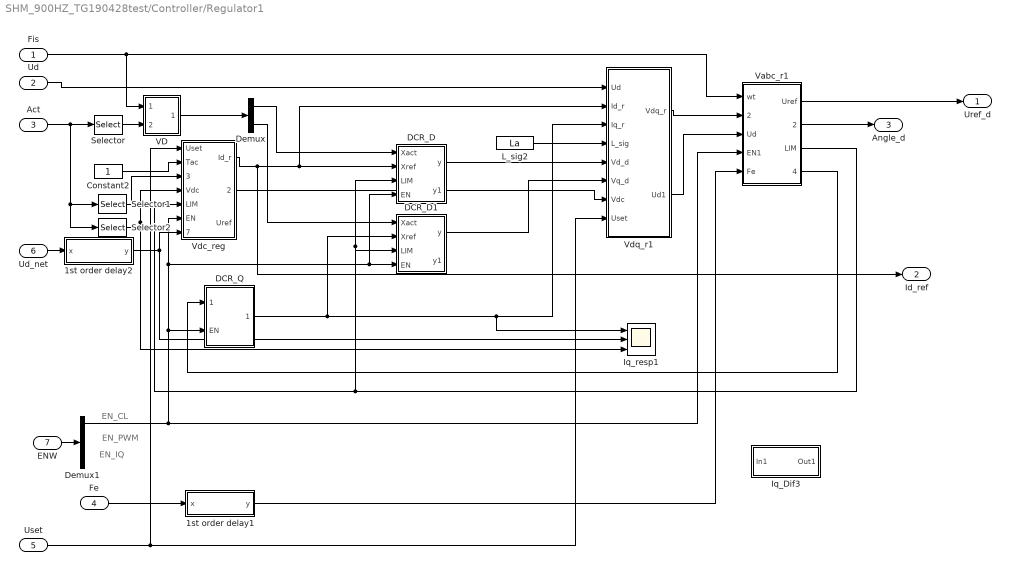
== system SHM_900HZ_TG190428test/Controller/Regulator1 ==
  note: EN_CL
  note: EN_PWM
  note: EN_IQ
  Fis : Inport
  Ud : Inport  Port=2
  Act : Inport  Port=3
  Fe : Inport  Port=4
  Uset : Inport  Port=5
  Ud_net : Inport  Port=6
  ENW : Inport  Port=7
  1st order delay1 : Subsystem
  1st order delay2 : Subsystem
  Constant2 : Constant
  DCR_D : Subsystem
  DCR_D1 : Subsystem
  DCR_Q : Subsystem
  Demux : Demux  Outputs=2
  Demux1 : Demux  Outputs=3
  Iq_Dif3 : Subsystem
  Iq_resp1 : Scope  NumInputPorts=3
      settings: YMin=-0.375~-0.3~-5  YMax=0.125~0.3~5  SaveName=ScopeData3  SampleInput=on  SampleTime=1E-4
  L_sig2 : Constant  Value=La
  Selector : Selector  InputPortWidth=10  IndexOptions=Index vector (dialog)  Indices=[8 9 10]  OutputSizes=1
  Selector1 : Selector  InputPortWidth=10  IndexOptions=Index vector (dialog)  Indices=4  OutputSizes=1
  Selector2 : Selector  InputPortWidth=10  IndexOptions=Index vector (dialog)  Indices=5  OutputSizes=1
  VD : Subsystem
  Vabc_r1 : Subsystem
  Vdc_reg : Subsystem
  Vdq_r1 : Subsystem
  Uref_d : Outport
  Id_ref : Outport  Port=2
  Angle_d : Outport  Port=3
  wires:
  Demux/1 -> DCR_D/1(Xact)
  Vdc_reg/1(Id_r) -> Vdq_r1/2(Id_r), DCR_D/2(Xref), Id_ref/1
  L_sig2/1 -> Vdq_r1/4(L_sig)
  Ud/1 -> Vdq_r1/1(Ud)
  Selector1/1 -> Vdc_reg/3(Idc_L)
  Fis/1 -> VD/1(Fis), Vabc_r1/1(wt)
  Vdq_r1/1(Vdq_r) -> Vabc_r1/2(Vdq_r)
  ENW/1 -> Demux1/1
  Selector/1 -> VD/2(Iac)
  VD/1(Idq) -> Demux/1
  Act/1 -> Selector/1, Selector2/1, Selector1/1
  Selector2/1 -> Vdc_reg/4(Vdc), Iq_resp1/3
  1st order delay1/1(y) -> Vabc_r1/5(Fe)
  Fe/1 -> 1st order delay1/1(x)
  Uset/1 -> Vdq_r1/8(Uset), Vdc_reg/1(Uset)
  Constant2/1 -> Vdc_reg/2(Tac)
  Vdq_r1/2(Ud1) -> Vabc_r1/3(Ud)
  Demux1/1 -> Vabc_r1/4(EN1), DCR_Q/2(EN), Vdc_reg/6(EN), DCR_D1/4(EN), DCR_D/4(EN)
  Vdc_reg/2(Vdc1) -> Vdq_r1/7(Vdc)
  Vabc_r1/2(Angle) -> Angle_d/1
  Vabc_r1/1(Uref) -> Uref_d/1
  DCR_D/1(y) -> Vdq_r1/5(Vd_d)
  Vabc_r1/3(LIM) -> DCR_D/3(LIM), DCR_D1/3(LIM), Vdc_reg/5(LIM)
  DCR_D1/1(y) -> Vdq_r1/6(Vq_d)
  Demux/2 -> DCR_D1/1(Xact)
  DCR_Q/1(Iq_ref) -> DCR_D1/2(Xref), Vdq_r1/3(Iq_r), Iq_resp1/1
  Vabc_r1/4(M_max) -> DCR_Q/1(M_max)
  Ud_net/1 -> 1st order delay2/1(x)
  1st order delay2/1(y) -> Vdc_reg/7(Ud_net), Iq_resp1/2

== system SHM_900HZ_TG190428test/Controller/Subsystem ==
  U_d : Inport
  Ang : Inport  Port=2
  EN : Inport  Port=3
  Constant1 : Constant  Value=180
  Constant2 : Constant  Value=[0 1 0 1 0 1 0 1 0 1 0 1 0 1 0 1 0 1 0]
  Direct Lookup Table (n-D) : LookupNDDirect  NumberOfTableDimensions=3  InputsSelectThisObjectFromTable=2-D Matrix  Table=SHM900  DiagnosticForOutOfRangeInput=Error
  Lookup Table Dynamic : simulink/Lookup Tables/Lookup Table Dynamic  LookUpMeth=Use Input Below  OutDataTypeStr=float('double')  OutputDataTypeScalingMode=Specify via dialog  OutDataType=float('double')  OutScaling=2^-10  DoSatur=off
  Math Function : Math  Operator=transpose  SaturateOnIntegerOverflow=on
  Math Function2 : Math  Operator=rem  SampleTime=Ts  SaturateOnIntegerOverflow=on
  PWM2 : Subsystem
  Relational Operator12 : RelationalOperator  OutDataTypeStr=boolean  SampleTime=Ts
  Puls : Outport
  wires:
  Direct Lookup Table (n-D)/1 -> Math Function/1
  Math Function/1 -> Lookup Table Dynamic/2
  Constant2/1 -> Lookup Table Dynamic/3
  Constant1/1 -> Math Function2/2, Relational Operator12/2
  Relational Operator12/1 -> PWM2/1(HW)
  Lookup Table Dynamic/1 -> PWM2/2(Real)
  Math Function2/1 -> Lookup Table Dynamic/1
  U_d/1 -> Direct Lookup Table (n-D)/1
  PWM2/1(P1) -> Puls/1
  EN/1 -> PWM2/3(EN)
  Ang/1 -> Relational Operator12/1, Math Function2/1

== system SHM_900HZ_TG190428test/Controller/Subsystem1 ==
  U_d : Inport
  Ang : Inport  Port=2
  EN : Inport  Port=3
  Constant1 : Constant  Value=180
  Constant2 : Constant  Value=[0 1 0 1 0 1 0 1 0 1 0 1 0 1 0 1 0 1 0]
  Direct Lookup Table (n-D) : LookupNDDirect  NumberOfTableDimensions=3  InputsSelectThisObjectFromTable=2-D Matrix  Table=SHM900  DiagnosticForOutOfRangeInput=Error
  Lookup Table Dynamic : simulink/Lookup Tables/Lookup Table Dynamic  LookUpMeth=Use Input Below  OutDataTypeStr=float('double')  OutputDataTypeScalingMode=Specify via dialog  OutDataType=float('double')  OutScaling=2^-10  DoSatur=off
  Math Function : Math  Operator=transpose  SaturateOnIntegerOverflow=on
  Math Function2 : Math  Operator=rem  SampleTime=Ts  SaturateOnIntegerOverflow=on
  PWM2 : Subsystem
  Relational Operator12 : RelationalOperator  OutDataTypeStr=boolean  SampleTime=Ts
  Puls : Outport
  wires:
  Ang/1 -> Math Function2/1, Relational Operator12/1
  EN/1 -> PWM2/3(EN)
  PWM2/1(P1) -> Puls/1
  U_d/1 -> Direct Lookup Table (n-D)/1
  Math Function2/1 -> Lookup Table Dynamic/1
  Lookup Table Dynamic/1 -> PWM2/2(Real)
  Relational Operator12/1 -> PWM2/1(HW)
  Constant1/1 -> Relational Operator12/2, Math Function2/2
  Constant2/1 -> Lookup Table Dynamic/3
  Math Function/1 -> Lookup Table Dynamic/2
  Direct Lookup Table (n-D)/1 -> Math Function/1

== system SHM_900HZ_TG190428test/Controller/Subsystem2 ==
  U_d : Inport
  Ang : Inport  Port=2
  EN : Inport  Port=3
  Constant1 : Constant  Value=180
  Constant2 : Constant  Value="[0 1 0 1 0 1 0 1 0 1 0 1 0 1  0 1 0 1 0]"
  Direct Lookup Table (n-D) : LookupNDDirect  NumberOfTableDimensions=3  InputsSelectThisObjectFromTable=2-D Matrix  Table=SHM900  DiagnosticForOutOfRangeInput=Error
  Lookup Table Dynamic : simulink/Lookup Tables/Lookup Table Dynamic  LookUpMeth=Use Input Below  OutDataTypeStr=float('double')  OutputDataTypeScalingMode=Specify via dialog  OutDataType=float('double')  OutScaling=2^-10  DoSatur=off
  Math Function : Math  Operator=transpose  SaturateOnIntegerOverflow=on
  Math Function2 : Math  Operator=rem  SampleTime=Ts  SaturateOnIntegerOverflow=on
  PWM2 : Subsystem
  Relational Operator12 : RelationalOperator  OutDataTypeStr=boolean  SampleTime=Ts
  Puls : Outport
  wires:
  Direct Lookup Table (n-D)/1 -> Math Function/1
  Math Function/1 -> Lookup Table Dynamic/2
  Constant2/1 -> Lookup Table Dynamic/3
  Constant1/1 -> Math Function2/2, Relational Operator12/2
  Relational Operator12/1 -> PWM2/1(HW)
  Lookup Table Dynamic/1 -> PWM2/2(Real)
  Math Function2/1 -> Lookup Table Dynamic/1
  U_d/1 -> Direct Lookup Table (n-D)/1
  PWM2/1(P1) -> Puls/1
  EN/1 -> PWM2/3(EN)
  Ang/1 -> Relational Operator12/1, Math Function2/1

== system SHM_900HZ_TG190428test/Controller/Subsystem3 ==
  Ang : Inport
  Constant : Constant  Value=360
  Constant3 : Constant  Value=360
  Constant4 : Constant  Value=0
  Math Function1 : Math  Operator=rem  SampleTime=Ts  SaturateOnIntegerOverflow=on
  Relational Operator1 : RelationalOperator  Operator=<  OutDataTypeStr=boolean  SampleTime=Ts
  Sum4 : Sum  SampleTime=Ts
  Switch1 : Switch  Threshold=0.5  ZeroCross=off  SampleTime=Ts
  Ang_ref : Outport
  wires:
  Constant/1 -> Math Function1/2
  Ang/1 -> Switch1/3, Sum4/2, Relational Operator1/1
  Constant3/1 -> Sum4/1
  Sum4/1 -> Switch1/1
  Switch1/1 -> Math Function1/1
  Relational Operator1/1 -> Switch1/2
  Constant4/1 -> Relational Operator1/2
  Math Function1/1 -> Ang_ref/1

== system SHM_900HZ_TG190428test/Controller/Subsystem4 ==
  Ang : Inport
  Constant : Constant  Value=360
  Constant3 : Constant  Value=360
  Constant4 : Constant  Value=0
  Math Function1 : Math  Operator=rem  SampleTime=Ts  SaturateOnIntegerOverflow=on
  Relational Operator1 : RelationalOperator  Operator=<  OutDataTypeStr=boolean  SampleTime=Ts
  Sum4 : Sum  SampleTime=Ts
  Switch1 : Switch  Threshold=0.5  ZeroCross=off  SampleTime=Ts
  Ang_ref : Outport
  wires:
  Math Function1/1 -> Ang_ref/1
  Constant4/1 -> Relational Operator1/2
  Relational Operator1/1 -> Switch1/2
  Switch1/1 -> Math Function1/1
  Sum4/1 -> Switch1/1
  Constant3/1 -> Sum4/1
  Ang/1 -> Relational Operator1/1, Sum4/2, Switch1/3
  Constant/1 -> Math Function1/2

== system SHM_900HZ_TG190428test/Controller/Subsystem5 ==
  Ang : Inport
  Constant : Constant  Value=360
  Constant3 : Constant  Value=360
  Constant4 : Constant  Value=0
  Math Function1 : Math  Operator=rem  SampleTime=Ts  SaturateOnIntegerOverflow=on
  Relational Operator1 : RelationalOperator  Operator=<  OutDataTypeStr=boolean  SampleTime=Ts
  Sum4 : Sum  SampleTime=Ts
  Switch1 : Switch  Threshold=0.5  ZeroCross=off  SampleTime=Ts
  Ang_ref : Outport
  wires:
  Constant/1 -> Math Function1/2
  Ang/1 -> Switch1/3, Sum4/2, Relational Operator1/1
  Constant3/1 -> Sum4/1
  Sum4/1 -> Switch1/1
  Switch1/1 -> Math Function1/1
  Relational Operator1/1 -> Switch1/2
  Constant4/1 -> Relational Operator1/2
  Math Function1/1 -> Ang_ref/1

== system SHM_900HZ_TG190428test/Controller/Uref_A ==
  Uref : Inport
  Constant1 : Constant  Value=0.8
  Constant4 : Constant  Value=0.001
  Divide : Product  Inputs=*/  SampleTime=TA
  Rounding Function : Rounding  SampleTime=TA
  Saturation : Saturate  UpperLimit=350  LowerLimit=0  ZeroCross=off
  Sum4 : Sum  Inputs=+-  SampleTime=TA
  Unit Delay4 : UnitDelay  SampleTime=TA
  Um : Outport
  wires:
  Constant1/1 -> Sum4/2
  Sum4/1 -> Divide/1
  Constant4/1 -> Divide/2
  Divide/1 -> Saturation/1
  Rounding Function/1 -> Unit Delay4/1
  Saturation/1 -> Rounding Function/1
  Uref/1 -> Sum4/1
  Unit Delay4/1 -> Um/1

== system SHM_900HZ_TG190428test/Controller/Uref_B ==
  Uref : Inport
  Constant1 : Constant  Value=0.8
  Constant4 : Constant  Value=0.001
  Divide : Product  Inputs=*/  SampleTime=TA
  Rounding Function : Rounding  SampleTime=TA
  Saturation : Saturate  UpperLimit=350  LowerLimit=0  ZeroCross=off
  Sum4 : Sum  Inputs=+-  SampleTime=TA
  Unit Delay4 : UnitDelay  SampleTime=TA
  Um : Outport
  wires:
  Unit Delay4/1 -> Um/1
  Uref/1 -> Sum4/1
  Saturation/1 -> Rounding Function/1
  Rounding Function/1 -> Unit Delay4/1
  Divide/1 -> Saturation/1
  Constant4/1 -> Divide/2
  Sum4/1 -> Divide/1
  Constant1/1 -> Sum4/2

== system SHM_900HZ_TG190428test/Controller/Uref_C ==
  Uref : Inport
  Constant1 : Constant  Value=0.8
  Constant4 : Constant  Value=0.001
  Divide : Product  Inputs=*/  SampleTime=TA
  Rounding Function : Rounding  SampleTime=TA
  Saturation : Saturate  UpperLimit=350  LowerLimit=0  ZeroCross=off
  Sum4 : Sum  Inputs=+-  SampleTime=TA
  Unit Delay4 : UnitDelay  SampleTime=TA
  Um : Outport
  wires:
  Constant1/1 -> Sum4/2
  Sum4/1 -> Divide/1
  Constant4/1 -> Divide/2
  Divide/1 -> Saturation/1
  Rounding Function/1 -> Unit Delay4/1
  Saturation/1 -> Rounding Function/1
  Uref/1 -> Sum4/1
  Unit Delay4/1 -> Um/1

== system SHM_900HZ_TG190428test/Controller/Uref_CM ==
  Uref_d : Inport
  Id_ref : Inport  Port=2
  Udc_sub : Inport  Port=3
  Abs : Abs  SampleTime=TA
  Constant3 : Constant  Value=0
  Constant5 : Constant
  Dead Zone : DeadZone  LowerValue=-0.01  UpperValue=0.01  SampleTime=TA  SaturateOnIntegerOverflow=on
  Product1 : Product  SampleTime=TA  RndMeth=Zero
  Product2 : Product  SampleTime=TA  RndMeth=Zero
  Product5 : Product  SampleTime=TA  RndMeth=Zero
  Relational Operator : RelationalOperator  OutDataTypeStr=boolean  SampleTime=TA
  Saturation : Saturate  UpperLimit=0.05  LowerLimit=0  SampleTime=TA
  Sum2 : Sum  SampleTime=TA
  Sum3 : Sum  Inputs=+-  SampleTime=TA
  V->pu6 : Gain  Gain=-1  SampleTime=TA  SaturateOnIntegerOverflow=on  OutDataTypeStr=Inherit: Same as input  ParamDataTypeStr=Inherit: Same as input
  Uref_H : Outport
  Uref_L : Outport  Port=2
  DIR : Outport  Port=3
  wires:
  Uref_d/1 -> Product1/1, Product2/1
  Id_ref/1 -> V->pu6/1
  Sum3/1 -> Product2/2
  Sum2/1 -> Product1/2
  Constant5/1 -> Sum3/1, Sum2/1
  Saturation/1 -> Sum3/2, Sum2/2
  Abs/1 -> Saturation/1
  Dead Zone/1 -> Abs/1
  Constant3/1 -> Relational Operator/2
  Product5/1 -> Relational Operator/1
  Udc_sub/1 -> Dead Zone/1, Product5/2
  V->pu6/1 -> Product5/1
  Relational Operator/1 -> DIR/1
  Product1/1 -> Uref_H/1
  Product2/1 -> Uref_L/1

== system SHM_900HZ_TG190428test/Measure1/Mean1 ==
  In : Inport
  Gain : Gain  Gain=1/Period  SaturateOnIntegerOverflow=on  OutDataTypeStr=Inherit: Same as input  ParamDataTypeStr=Inherit: Same as input
  Integrator : Integrator
  Sum : Sum  Inputs=+-  SaturateOnIntegerOverflow=on  InputSameDT=on  OutDataTypeStr=Inherit: Same as first input
  Transport Delay : TransportDelay  DelayTime=Period  BufferSize=buf
  Out : Outport
  wires:
  Sum/1 -> Gain/1
  Transport Delay/1 -> Sum/2
  In/1 -> Integrator/1
  Integrator/1 -> Transport Delay/1, Sum/1
  Gain/1 -> Out/1

== system SHM_900HZ_TG190428test/Measure1/Mean2 ==
  In : Inport
  Gain : Gain  Gain=1/Period  SaturateOnIntegerOverflow=on  OutDataTypeStr=Inherit: Same as input  ParamDataTypeStr=Inherit: Same as input
  Integrator : Integrator
  Sum : Sum  Inputs=+-  SaturateOnIntegerOverflow=on  InputSameDT=on  OutDataTypeStr=Inherit: Same as first input
  Transport Delay : TransportDelay  DelayTime=Period  BufferSize=buf
  Out : Outport
  wires:
  Gain/1 -> Out/1
  Integrator/1 -> Sum/1, Transport Delay/1
  In/1 -> Integrator/1
  Transport Delay/1 -> Sum/2
  Sum/1 -> Gain/1

== system SHM_900HZ_TG190428test/Measure1/Mean3 ==
  In : Inport
  Gain : Gain  Gain=1/Period  SaturateOnIntegerOverflow=on  OutDataTypeStr=Inherit: Same as input  ParamDataTypeStr=Inherit: Same as input
  Integrator : Integrator
  Sum : Sum  Inputs=+-  SaturateOnIntegerOverflow=on  InputSameDT=on  OutDataTypeStr=Inherit: Same as first input
  Transport Delay : TransportDelay  DelayTime=Period  BufferSize=buf
  Out : Outport
  wires:
  Sum/1 -> Gain/1
  Transport Delay/1 -> Sum/2
  In/1 -> Integrator/1
  Integrator/1 -> Transport Delay/1, Sum/1
  Gain/1 -> Out/1

== system SHM_900HZ_TG190428test/Measure1/Mean5 ==
  In : Inport
  Gain : Gain  Gain=1/Period  SaturateOnIntegerOverflow=on  OutDataTypeStr=Inherit: Same as input  ParamDataTypeStr=Inherit: Same as input
  Integrator : Integrator
  Sum : Sum  Inputs=+-  SaturateOnIntegerOverflow=on  InputSameDT=on  OutDataTypeStr=Inherit: Same as first input
  Transport Delay : TransportDelay  DelayTime=Period  BufferSize=buf
  Out : Outport
  wires:
  Gain/1 -> Out/1
  Integrator/1 -> Sum/1, Transport Delay/1
  In/1 -> Integrator/1
  Transport Delay/1 -> Sum/2
  Sum/1 -> Gain/1

== system SHM_900HZ_TG190428test/Measure1/Mean6 ==
  In : Inport
  Gain : Gain  Gain=1/Period  SaturateOnIntegerOverflow=on  OutDataTypeStr=Inherit: Same as input  ParamDataTypeStr=Inherit: Same as input
  Integrator : Integrator
  Sum : Sum  Inputs=+-  SaturateOnIntegerOverflow=on  InputSameDT=on  OutDataTypeStr=Inherit: Same as first input
  Transport Delay : TransportDelay  DelayTime=Period  BufferSize=buf
  Out : Outport
  wires:
  Sum/1 -> Gain/1
  Transport Delay/1 -> Sum/2
  In/1 -> Integrator/1
  Integrator/1 -> Transport Delay/1, Sum/1
  Gain/1 -> Out/1

== system SHM_900HZ_TG190428test/Measure1/Mean7 ==
  In : Inport
  Gain : Gain  Gain=1/Period  SaturateOnIntegerOverflow=on  OutDataTypeStr=Inherit: Same as input  ParamDataTypeStr=Inherit: Same as input
  Integrator : Integrator
  Sum : Sum  Inputs=+-  SaturateOnIntegerOverflow=on  InputSameDT=on  OutDataTypeStr=Inherit: Same as first input
  Transport Delay : TransportDelay  DelayTime=Period  BufferSize=buf
  Out : Outport
  wires:
  Gain/1 -> Out/1
  Integrator/1 -> Sum/1, Transport Delay/1
  In/1 -> Integrator/1
  Transport Delay/1 -> Sum/2
  Sum/1 -> Gain/1

== system SHM_900HZ_TG190428test/Subsystem1/POWER ==
  K_U : Inport
  Add : Sum
  Add1 : Sum
  Add2 : Sum
  Controlled Voltage Source : powerlib/Electrical Sources/Controlled Voltage Source  SystemSampleTime=-1  Initialize=on  Source_Type=AC  Amplitude=0  Phase=0  Frequency=0  Measurements=None
  Controlled Voltage Source1 : powerlib/Electrical Sources/Controlled Voltage Source  SystemSampleTime=-1  Initialize=on  Source_Type=AC  Amplitude=0  Phase=0  Frequency=0  Measurements=None
  Controlled Voltage Source2 : powerlib/Electrical Sources/Controlled Voltage Source  SystemSampleTime=-1  Initialize=on  Source_Type=AC  Amplitude=0  Phase=0  Frequency=0  Measurements=None
  Product : Product  RndMeth=Zero
  Product1 : Product  RndMeth=Zero
  Product2 : Product  RndMeth=Zero
  UA : Sin  Amplitude=UL*sqrt(2/3)*1000  Frequency=100*pi  SampleTime=0
  UB : Sin  Amplitude=UL*sqrt(2/3)*1000  Frequency=100*pi  Phase=-2/3*pi  SampleTime=0
  UC : Sin  Amplitude=UL*sqrt(2/3)*1000  Frequency=100*pi  Phase=2/3*pi  SampleTime=0
  UthA : Sin  Amplitude=UL*sqrt(2/3)*Uth*1000  Frequency=100*TH*pi  SampleTime=0
  UthB : Sin  Amplitude=UL*sqrt(2/3)*Uth*1000  Frequency=100*TH*pi  Phase=-2/3*pi  SampleTime=0
  UthC : Sin  Amplitude=UL*sqrt(2/3)*Uth*1000  Frequency=100*TH*pi  Phase=2/3*pi  SampleTime=0
  UA1 : PMIOPort  Port=1  Side=Right
  UB1 : PMIOPort  Port=2  Side=Right
  UC1 : PMIOPort  Port=3  Side=Right
  wires:
  UA/1 -> Add/1
  UB/1 -> Add1/1
  UC/1 -> Add2/1
  UthC/1 -> Add2/2
  UthB/1 -> Add1/2
  UthA/1 -> Add/2
  Add/1 -> Product/1
  Product/1 -> Controlled Voltage Source/1
  Add1/1 -> Product1/1
  Product1/1 -> Controlled Voltage Source1/1
  Add2/1 -> Product2/1
  Product2/1 -> Controlled Voltage Source2/1
  K_U/1 -> Product/2, Product1/2, Product2/2
  connections:
  UA1/RConn1 -- Controlled Voltage Source/RConn1
  UB1/RConn1 -- Controlled Voltage Source1/RConn1
  UC1/RConn1 -- Controlled Voltage Source2/RConn1
  Controlled Voltage Source/LConn1 -- Controlled Voltage Source2/LConn1 -- Controlled Voltage Source1/LConn1

== system SHM_900HZ_TG190428test/Subsystem1/V-I_M1 ==
  CM : powerlib/Measurements/Current Measurement  SystemSampleTime=-1  PhasorSimulation=off  OutputType=Complex  PSBequivalent=0
  CM1 : powerlib/Measurements/Current Measurement  SystemSampleTime=-1  PhasorSimulation=off  OutputType=Complex  PSBequivalent=0
  CM2 : powerlib/Measurements/Current Measurement  SystemSampleTime=-1  PhasorSimulation=off  OutputType=Complex  PSBequivalent=0
  Mux4 : Mux  Inputs=6
  Voltage Measurement1 : powerlib/Measurements/Voltage Measurement  SystemSampleTime=-1  PhasorSimulation=off  OutputType=Complex  PSBequivalent=0
  Voltage Measurement3 : powerlib/Measurements/Voltage Measurement  SystemSampleTime=-1  PhasorSimulation=off  OutputType=Complex  PSBequivalent=0
  Voltage Measurement4 : powerlib/Measurements/Voltage Measurement  SystemSampleTime=-1  PhasorSimulation=off  OutputType=Complex  PSBequivalent=0
  A1 : PMIOPort  Port=1  Side=Left
  B1 : PMIOPort  Port=2  Side=Left
  C1 : PMIOPort  Port=3  Side=Left
  A2 : PMIOPort  Port=4  Side=Right
  B2 : PMIOPort  Port=5  Side=Right
  C2 : PMIOPort  Port=6  Side=Right
  V-I : Outport
  wires:
  Voltage Measurement1/1 -> Mux4/1  "Vab"
  Voltage Measurement3/1 -> Mux4/2
  Voltage Measurement4/1 -> Mux4/3
  Mux4/1 -> V-I/1
  CM/1 -> Mux4/4
  CM2/1 -> Mux4/5
  CM1/1 -> Mux4/6
  connections:
  A1/RConn1 -- CM/LConn1 -- Voltage Measurement4/LConn2 -- Voltage Measurement1/LConn1
  C1/RConn1 -- Voltage Measurement3/LConn2 -- Voltage Measurement4/LConn1 -- CM1/LConn1
  B1/RConn1 -- CM2/LConn1 -- Voltage Measurement1/LConn2 -- Voltage Measurement3/LConn1
  A2/RConn1 -- CM/RConn1
  B2/RConn1 -- CM2/RConn1
  C2/RConn1 -- CM1/RConn1

== system SHM_900HZ_TG190428test/Controller/PLL/1st order delay ==
  x : Inport
  Kd_1 : Gain  Gain=TA/(T1*sqrt(3)/pi+TA*0.5)  SampleTime=TA
  Kd_2 : Gain  Gain=0.5  SampleTime=TA
  Sum1 : Sum  SampleTime=TA
  Sum4 : Sum  Inputs=+-  SampleTime=TA
  Sum6 : Sum  SampleTime=TA
  Unit Delay1 : UnitDelay  SampleTime=TA
  y : Outport
  wires:
  x/1 -> Sum4/1
  Unit Delay1/1 -> Sum6/2, Sum4/2, Sum1/2
  Sum6/1 -> Unit Delay1/1, Sum1/1
  Kd_1/1 -> Sum6/1
  Sum4/1 -> Kd_1/1
  Sum1/1 -> Kd_2/1
  Kd_2/1 -> y/1

== system SHM_900HZ_TG190428test/Controller/PLL/INT1 ==
  Freq : Inport
  Add : Sum  SampleTime=TA
  Constant2 : Constant
  Gain6 : Gain  Gain=2*pi  SampleTime=TA
  Math Function1 : Math  Operator=rem  SampleTime=TA  SaturateOnIntegerOverflow=on
  Unit Delay2 : UnitDelay  SampleTime=TA
  k1 : Gain  Gain=TA*fn  SampleTime=TA
  Angle : Outport
  wires:
  Freq/1 -> k1/1
  k1/1 -> Add/1
  Add/1 -> Math Function1/1
  Math Function1/1 -> Unit Delay2/1, Gain6/1
  Unit Delay2/1 -> Add/2
  Constant2/1 -> Math Function1/2
  Gain6/1 -> Angle/1
